simulink model "Coupling"  (R2024b)
settings: Solver=VariableStepAuto  StartTime=0.0  StopTime=0.2  RelTol=1e-3
settings Model: Creator=Zohaib  LastModifiedBy=Zohaib

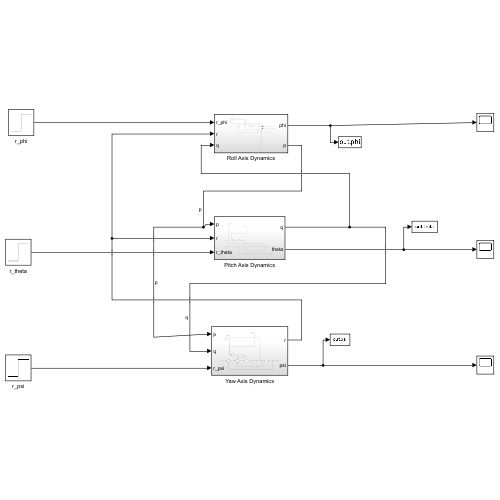
[thumbnail: Simulink's stored preview of the top-level diagram]
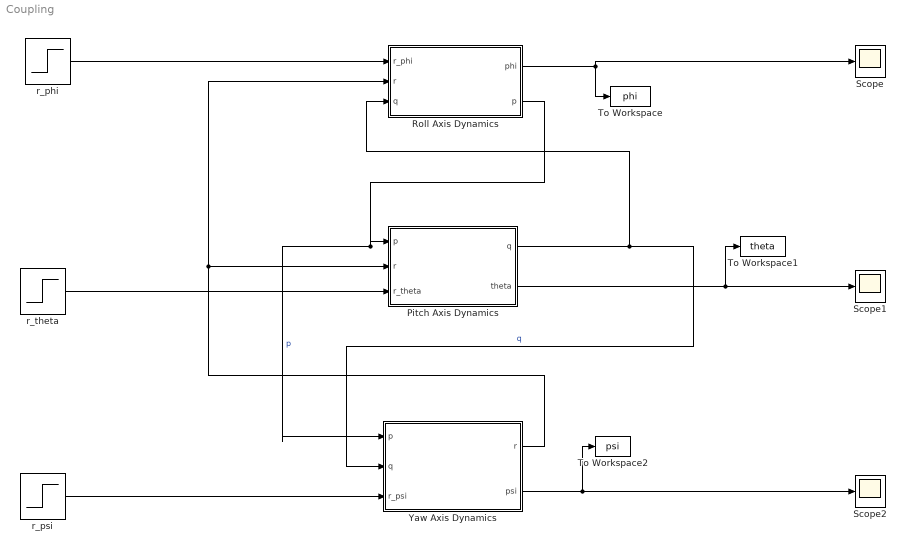
== system Coupling ==
  Pitch Axis Dynamics : Subsystem
  Roll Axis Dynamics : Subsystem
  Scope : Scope
  Scope1 : Scope
  Scope2 : Scope
  To Workspace : ToWorkspace  VariableName=phi  SaveFormat=Timeseries  SampleTime=-1
  To Workspace1 : ToWorkspace  VariableName=theta  SaveFormat=Timeseries  SampleTime=-1
  To Workspace2 : ToWorkspace  VariableName=psi  SaveFormat=Timeseries  SampleTime=-1
  Yaw Axis Dynamics : Subsystem
  r_phi : Step  Time=0  After=1.0001  SampleTime=0
  r_psi : Step  Time=0  After=1.0001  SampleTime=0
  r_theta : Step  Time=0  After=1.0001  SampleTime=0
  wires:
  r_phi/1 -> Roll Axis Dynamics/1(r_phi)
  Roll Axis Dynamics/1(phi) -> To Workspace/1, Scope/1
  Roll Axis Dynamics/2(p) -> Yaw Axis Dynamics/1(p), Pitch Axis Dynamics/1(p)  "p"
  r_theta/1 -> Pitch Axis Dynamics/3(r_theta)
  Pitch Axis Dynamics/1(q) -> Yaw Axis Dynamics/2(q), Roll Axis Dynamics/3(q)  "q"
  Pitch Axis Dynamics/2(theta) -> To Workspace1/1, Scope1/1
  Yaw Axis Dynamics/1(r) -> Roll Axis Dynamics/2(r), Pitch Axis Dynamics/2(r)
  r_psi/1 -> Yaw Axis Dynamics/3(r_psi)
  Yaw Axis Dynamics/2(psi) -> To Workspace2/1, Scope2/1

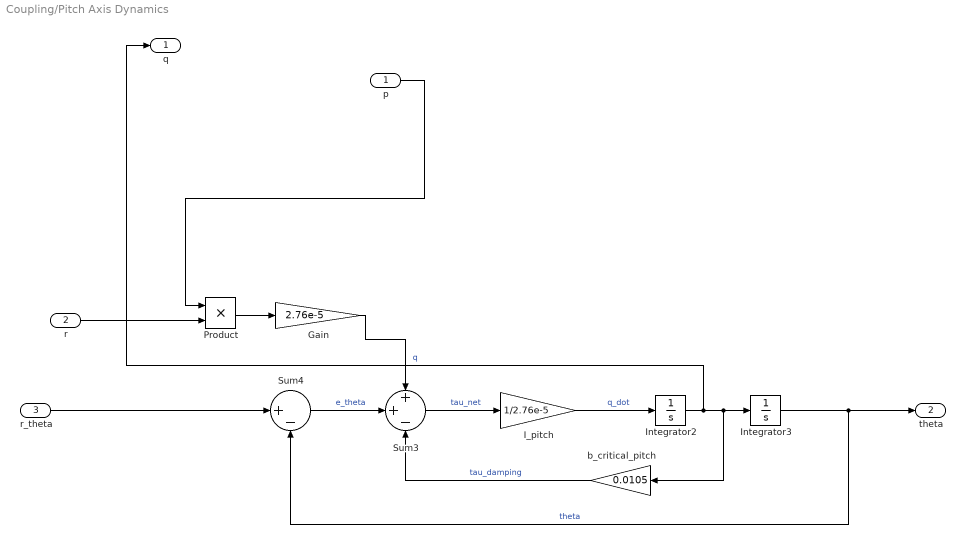
== system Coupling/Pitch Axis Dynamics ==
  p : Inport
  r : Inport  Port=2
  r_theta : Inport  Port=3
  Gain : Gain  Gain=2.76e-5
  I_pitch : Gain  Gain=1/2.76e-5
  Integrator2 : Integrator
  Integrator3 : Integrator
  Product : Product
  Sum3 : Sum  Inputs=++-
  Sum4 : Sum  Inputs=|+-
  b_critical_pitch : Gain  Gain=0.0105
  q : Outport
  theta : Outport  Port=2
  wires:
  r/1 -> Product/2
  Integrator2/1 -> q/1, b_critical_pitch/1, Integrator3/1  "q"
  b_critical_pitch/1 -> Sum3/3  "tau_damping"
  Sum3/1 -> I_pitch/1  "tau_net"
  Product/1 -> Gain/1
  Sum4/1 -> Sum3/2  "e_theta"
  Gain/1 -> Sum3/1
  I_pitch/1 -> Integrator2/1  "q_dot"
  Integrator3/1 -> theta/1, Sum4/2  "theta"
  p/1 -> Product/1
  r_theta/1 -> Sum4/1

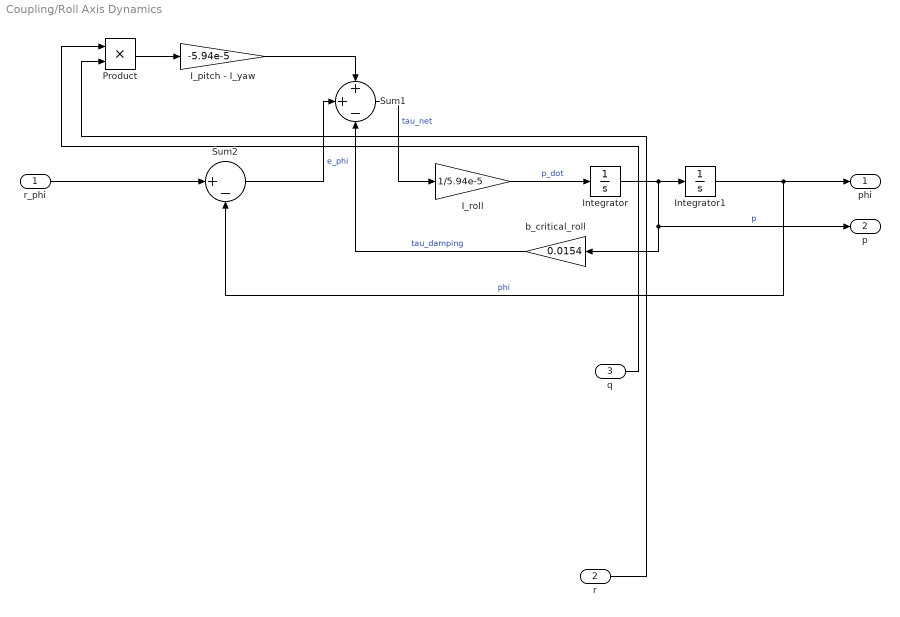
== system Coupling/Roll Axis Dynamics ==
  r_phi : Inport
  r : Inport  Port=2
  q : Inport  Port=3
  I_pitch - I_yaw : Gain  Gain=-5.94e-5
  I_roll : Gain  Gain=1/5.94e-5
  Integrator : Integrator
  Integrator1 : Integrator
  Product : Product
  Sum1 : Sum  Inputs=++-
  Sum2 : Sum  Inputs=|+-
  b_critical_roll : Gain  Gain=0.0154
  phi : Outport
  p : Outport  Port=2
  wires:
  I_pitch - I_yaw/1 -> Sum1/1
  b_critical_roll/1 -> Sum1/3  "tau_damping"
  Integrator1/1 -> phi/1, Sum2/2  "phi"
  Sum2/1 -> Sum1/2  "e_phi"
  Product/1 -> I_pitch - I_yaw/1
  I_roll/1 -> Integrator/1  "p_dot"
  Integrator/1 -> p/1, b_critical_roll/1, Integrator1/1  "p"
  Sum1/1 -> I_roll/1  "tau_net"
  r/1 -> Product/2
  q/1 -> Product/1
  r_phi/1 -> Sum2/1

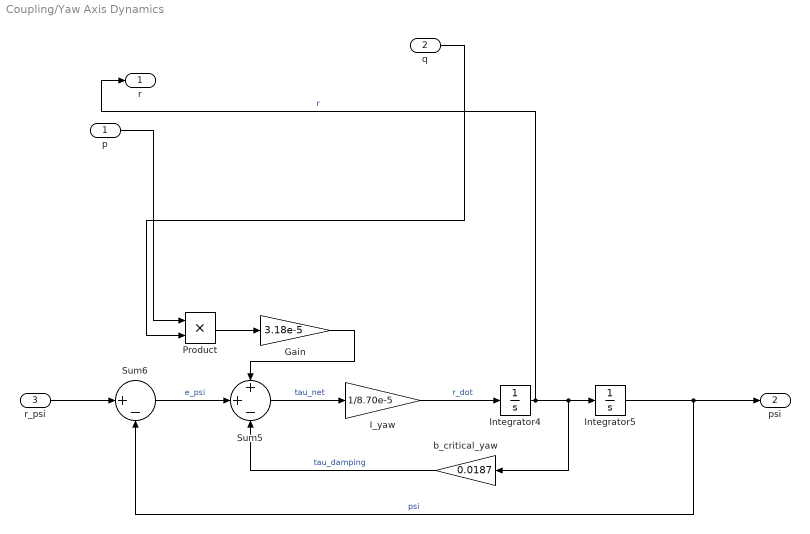
== system Coupling/Yaw Axis Dynamics ==
  p : Inport
  q : Inport  Port=2
  r_psi : Inport  Port=3
  Gain : Gain  Gain=3.18e-5
  I_yaw : Gain  Gain=1/8.70e-5
  Integrator4 : Integrator
  Integrator5 : Integrator
  Product : Product
  Sum5 : Sum  Inputs=++-
  Sum6 : Sum  Inputs=|+-
  b_critical_yaw : Gain  Gain=0.0187
  r : Outport
  psi : Outport  Port=2
  wires:
  Sum6/1 -> Sum5/2  "e_psi"
  Gain/1 -> Sum5/1
  Integrator5/1 -> psi/1, Sum6/2  "psi"
  I_yaw/1 -> Integrator4/1  "r_dot"
  Integrator4/1 -> r/1, b_critical_yaw/1, Integrator5/1  "r"
  q/1 -> Product/2
  b_critical_yaw/1 -> Sum5/3  "tau_damping"
  Product/1 -> Gain/1
  r_psi/1 -> Sum6/1
  p/1 -> Product/1
  Sum5/1 -> I_yaw/1  "tau_net"
